simulink model "HMC"  (R2026a)
settings: Solver=ode1  StopTime=inf  FixedStep=0.0001
PreLoadFcn:
  | %load('C:\Users\bme_master\Desktop\mot\mot_6_deneme.mat')
  | 
  | 
  | %load('C:\Users\bme_master\Desktop\mot\PRE_G''s.mat')
PostLoadFcn:
  | , if any(exist('dsrtsu_mdlpostloadfcn', 'file') ~= 0), dsrtsu_mdlpostloadfcn('Execute', bdroot); end,
InitFcn:
  | %motor_control_init_m
  | %clear all
  | %close all
  | %clc
  | b=1e-8
  | StepSize = 1e-4;
  | N=1e-17;
  | 
  | VLV_0 =0;%120; %120
  | VA_0 = 0;%300; %300
  | VRV_0 = 0;%130;
  | VP_0 = 0;%500;
  | VLA_0 = 0;%20;
  | VV_0=5000;
  | VRA_0=0;
  | 
  | 
  | QLV_0 = 0;
  | QLA_0 = 0;
  | QP_0 = 0;
  | 
  | bh = 0;
  | th =0;
  | 
  | X_0 = [VLV_0 VA_0 VV_0 VP_0  VLA_0  VRA_0 VRV_0];
  | 
  | 
  | V0 = 10;
  | 
  | K1=.0004;%0.0001
  | K2=0.0009;%0.0009
  | KA=1;%1
  | C1=0.000000003;%0.0000003
  | lambda=6000;%3000
  | X_00 = [VLV_0 VA_0 VV_0 VRV_0];
  | 
  | r2 = 0.05/2;
  | A2 = pi*r2^2;
  | h2 = 0.63;
  | V2 = A2*h2;
  | 
  | 
  | r3 = 0.05/2;
  | A3 = pi*r3^2;
  | h3 = 0.63;
  | V3 = A3*h3;
  | 
  | 
  | rho = 997;
  | gg = 9.81;
  | %
  | init_min=0;
  | init_max=0;
  | %
  | PWM_Period =  StepSize;
  | PWM_Period_g1 = PWM_Period;
  | PWM_Period_g2 =PWM_Period;
  | PWM_Period_g3 = PWM_Period;
  | PWM_Period_g4 = PWM_Period;
  | PWM_Period_g5 = PWM_Period;
  | ... (+158 lines)
undefined symbols (not defined in the file or in its folder): Continuous, DiscIntNeverNeededParam, Time
libraries: powerlib_meascontrol x19, simulink x15, rti1202lib_adc_class1 x11, cstblocks x10, rti1202lib_dio_class1 x8, dspstat3 x3, rti1202lib_dac_class1 x1, dspswit3 x1, ctrlSharedLib x1, slpidlib x1, dsparch4 x1
(part 5 of 5)

== system HMC/Reference CVSs/eRV/RV_e_min/c_RV/PID ==
  s : Inport
  LTI System : cstblocks/LTI System  sys=tfa  IC=[]
  PID Controller : simulink/Continuous/PID Controller  Controller=PID  Form=Parallel  TimeDomain=Continuous-time  SampleTime=-1  IntegratorMethod=Forward Euler  FilterMethod=Forward Euler  ControllerParametersSource=internal  P=0  I=0.336541519886425  D=0  UseFilter=on  N=100  TunerSelectOption=Transfer Function Based (PID Tuner App)  InitialConditionSource=internal  InitialConditionForIntegrator=0  InitialConditionForFilter=0  DifferentiatorICPrevScaledInput=0  ExternalReset=none  TrackingMode=off  Kt=1  LimitOutput=off  UpperSaturationLimit=inf  LowerSaturationLimit=-inf  LinearizeAsGain=on  AntiWindupMode=none  Kb=1  POutMin=[]  POutMax=[]  IOutMin=[]  IOutMax=[]  DOutMin=[]  DOutMax=[]  NOutMin=[]  NOutMax=[]  SumOutMin=[]  SumOutMax=[]  SaturationOutMin=[]  SaturationOutMax=[]  PParamMin=[]  PParamMax=[]  IParamMin=[]  IParamMax=[]  DParamMin=[]  DParamMax=[]  NParamMin=[]  NParamMax=[]  KbParamMin=[]  KbParamMax=[]  KtParamMin=[]  KtParamMax=[]  KbOutMin=[]  KbOutMax=[]  KtOutMin=[]  KtOutMax=[]  IntegratorOutMin=[]  IntegratorOutMax=[]  FilterOutMin=[]  FilterOutMax=[]  SumI1OutMin=[]  SumI1OutMax=[]  SumI2OutMin=[]  SumI2OutMax=[]  SumI3OutMin=[]  SumI3OutMax=[]  SumI4OutMin=[]  SumI4OutMax=[]  SumDOutMin=[]  SumDOutMax=[]  DifferentiatorOutMin=[]  DifferentiatorOutMax=[]  FilterDiffOutCoefMin=[]  FilterDiffOutCoefMax=[]  ReciprocalOutMin=[]  ReciprocalOutMax=[]  SumDenOutMin=[]  SumDenOutMax=[]  SumNumOutMin=[]  SumNumOutMax=[]  DivideOutMin=[]  DivideOutMax=[]  IntegratorContinuousStateAttributes=''  IntegratorStateMustResolveToSignalObject=off  IntegratorRTWStateStorageClass=Auto  FilterContinuousStateAttributes=''  FilterStateMustResolveToSignalObject=off  FilterRTWStateStorageClass=Auto  ParallelPVariant=InternalParameters  IdealPVariant=Disabled  IVariant=InternalParameters  DVariant=InternalParameters  IntegratorVariant=Continuous  SatVariant=Disabled  AWVariant=Passthrough  PCopyVariant=Disabled  TRVariant=Disabled  FdbkBlocksVariant=Forward  IdealPFdbkVariant=Disabled  SatFdbkVariant=Disabled  DerivativeFilterVariant=ContFilter  NVariant=InternalParameters  NCopyVariant=Disabled  FilterICVariant=InternalICsFilter  IntegratorICVariant=InternalICs  ExternalResetVariant=Disabled  TRSumVariant=Passthrough  SumFdbkVariant=Disabled  SumVariant=Sum_PID
  Sum1 : Sum  Inputs=|+-
  To Workspace : ToWorkspace  VariableName=input  SampleTime=-1
  To Workspace1 : ToWorkspace  VariableName=output  SampleTime=-1
  E : Outport  VectorParamsAs1DForOutWhenUnconnected=off
  wires:
  LTI System/1 -> To Workspace1/1, E/1, Sum1/2
  Sum1/1 -> PID Controller/1
  s/1 -> Sum1/1
  PID Controller/1 -> LTI System/1, To Workspace/1

== system HMC/Reference CVSs/eRV/RV_e_min/real_c_RV/PID ==
  s : Inport
  LTI System : cstblocks/LTI System  sys=tfa  IC=[]
  PID Controller : simulink/Continuous/PID Controller  Controller=PID  Form=Parallel  TimeDomain=Continuous-time  SampleTime=-1  IntegratorMethod=Forward Euler  FilterMethod=Forward Euler  ControllerParametersSource=internal  P=0  I=0.336541519886425  D=0  UseFilter=on  N=100  TunerSelectOption=Transfer Function Based (PID Tuner App)  InitialConditionSource=internal  InitialConditionForIntegrator=0  InitialConditionForFilter=0  DifferentiatorICPrevScaledInput=0  ExternalReset=none  TrackingMode=off  Kt=1  LimitOutput=off  UpperSaturationLimit=inf  LowerSaturationLimit=-inf  LinearizeAsGain=on  AntiWindupMode=none  Kb=1  POutMin=[]  POutMax=[]  IOutMin=[]  IOutMax=[]  DOutMin=[]  DOutMax=[]  NOutMin=[]  NOutMax=[]  SumOutMin=[]  SumOutMax=[]  SaturationOutMin=[]  SaturationOutMax=[]  PParamMin=[]  PParamMax=[]  IParamMin=[]  IParamMax=[]  DParamMin=[]  DParamMax=[]  NParamMin=[]  NParamMax=[]  KbParamMin=[]  KbParamMax=[]  KtParamMin=[]  KtParamMax=[]  KbOutMin=[]  KbOutMax=[]  KtOutMin=[]  KtOutMax=[]  IntegratorOutMin=[]  IntegratorOutMax=[]  FilterOutMin=[]  FilterOutMax=[]  SumI1OutMin=[]  SumI1OutMax=[]  SumI2OutMin=[]  SumI2OutMax=[]  SumI3OutMin=[]  SumI3OutMax=[]  SumI4OutMin=[]  SumI4OutMax=[]  SumDOutMin=[]  SumDOutMax=[]  DifferentiatorOutMin=[]  DifferentiatorOutMax=[]  FilterDiffOutCoefMin=[]  FilterDiffOutCoefMax=[]  ReciprocalOutMin=[]  ReciprocalOutMax=[]  SumDenOutMin=[]  SumDenOutMax=[]  SumNumOutMin=[]  SumNumOutMax=[]  DivideOutMin=[]  DivideOutMax=[]  IntegratorContinuousStateAttributes=''  IntegratorStateMustResolveToSignalObject=off  IntegratorRTWStateStorageClass=Auto  FilterContinuousStateAttributes=''  FilterStateMustResolveToSignalObject=off  FilterRTWStateStorageClass=Auto  ParallelPVariant=InternalParameters  IdealPVariant=Disabled  IVariant=InternalParameters  DVariant=InternalParameters  IntegratorVariant=Continuous  SatVariant=Disabled  AWVariant=Passthrough  PCopyVariant=Disabled  TRVariant=Disabled  FdbkBlocksVariant=Forward  IdealPFdbkVariant=Disabled  SatFdbkVariant=Disabled  DerivativeFilterVariant=ContFilter  NVariant=InternalParameters  NCopyVariant=Disabled  FilterICVariant=InternalICsFilter  IntegratorICVariant=InternalICs  ExternalResetVariant=Disabled  TRSumVariant=Passthrough  SumFdbkVariant=Disabled  SumVariant=Sum_PID
  Sum1 : Sum  Inputs=|+-
  To Workspace : ToWorkspace  VariableName=input  SampleTime=-1
  To Workspace1 : ToWorkspace  VariableName=output  SampleTime=-1
  E : Outport  VectorParamsAs1DForOutWhenUnconnected=off
  wires:
  PID Controller/1 -> To Workspace/1, LTI System/1
  s/1 -> Sum1/1
  Sum1/1 -> PID Controller/1
  LTI System/1 -> Sum1/2, E/1, To Workspace1/1

== system HMC/IBS_LVAD/Subsystem1/Subsystem/eLV1/LV_e_min/Subsystem1 ==
  note: y = 0,0446x 2 - 6,3542x + 365,75
      | R² = 1
  Add18 : Sum
  Add19 : Sum
  Constant20 : Constant  Value=365.75
  Gain2 : Gain  Gain=0.0446
  Gain3 : Gain  Gain=- 6.3542
  Product15 : Product
  C_LV : Outport
  wires:
  Add18/1 -> Add19/1
  Gain3/1 -> Add18/2
  Product15/1 -> Gain2/1
  Constant20/1 -> Add19/2
  Gain2/1 -> Add18/1
  [HR] -> Product15/1, Product15/2, Gain3/1
  Add19/1 -> C_LV/1

== system HMC/IBS_LVAD/Subsystem1/Subsystem/eLV1/LV_e_min/Subsystem2 ==
  note: y = 0,0108x 2 - 4,2917x + 398,5
      | R² = 1
  note: y = 0,0011x 2 - 0,4292x + 39,85
      | R² = 1
  note: y = -0,0175x 2 + 5,625x - 264,5
      | R² = 1
  Add18 : Sum
  Add19 : Sum
  Constant20 : Constant  Value=398.5
  Gain : Gain  Gain=1/10000
  Gain2 : Gain  Gain=0.0108
  Gain3 : Gain  Gain=-4.2917
  Product15 : Product
  Scope : Scope
      settings: ActiveDisplayYMinimum=-0.00112  ActiveDisplayYMaximum=0.02012  DataLoggingVariableName=ScopeData2
  B_LV : Outport
  wires:
  Add18/1 -> Add19/1
  Gain3/1 -> Add18/2
  Product15/1 -> Gain2/1
  Constant20/1 -> Add19/2
  Gain2/1 -> Add18/1
  [HR] -> Product15/1, Product15/2, Gain3/1
  Add19/1 -> Gain/1
  Gain/1 -> Scope/1, B_LV/1

== system HMC/IBS_LVAD/Subsystem1/Subsystem/eLV1/LV_e_min/resting ==
  note: y = -4,3333x + 440
  Add19 : Sum
  Constant20 : Constant  Value=440
  Gain : Gain  Gain=1/10000
  Gain3 : Gain  Gain=-4.3333
  Scope : Scope
      settings: ActiveDisplayYMinimum=-0.00112  ActiveDisplayYMaximum=0.02012  DataLoggingVariableName=ScopeData2
  B_LV : Outport
  wires:
  Gain/1 -> B_LV/1, Scope/1
  Add19/1 -> Gain/1
  [insan] -> Gain3/1
  Constant20/1 -> Add19/2
  Gain3/1 -> Add19/1

== system HMC/IBS_LVAD/Subsystem1/Subsystem/eLV1/eLV1/PID ==
  s : Inport
  LTI System : cstblocks/LTI System  sys=tfa  IC=[]
  PID Controller : simulink/Continuous/PID Controller  Controller=PID  Form=Parallel  TimeDomain=Continuous-time  SampleTime=-1  IntegratorMethod=Forward Euler  FilterMethod=Forward Euler  ControllerParametersSource=internal  P=0  I=0.336541519886425  D=0  UseFilter=on  N=100  TunerSelectOption=Transfer Function Based (PID Tuner App)  InitialConditionSource=internal  InitialConditionForIntegrator=0  InitialConditionForFilter=0  DifferentiatorICPrevScaledInput=0  ExternalReset=none  TrackingMode=off  Kt=1  LimitOutput=off  UpperSaturationLimit=inf  LowerSaturationLimit=-inf  LinearizeAsGain=on  AntiWindupMode=none  Kb=1  POutMin=[]  POutMax=[]  IOutMin=[]  IOutMax=[]  DOutMin=[]  DOutMax=[]  NOutMin=[]  NOutMax=[]  SumOutMin=[]  SumOutMax=[]  SaturationOutMin=[]  SaturationOutMax=[]  PParamMin=[]  PParamMax=[]  IParamMin=[]  IParamMax=[]  DParamMin=[]  DParamMax=[]  NParamMin=[]  NParamMax=[]  KbParamMin=[]  KbParamMax=[]  KtParamMin=[]  KtParamMax=[]  KbOutMin=[]  KbOutMax=[]  KtOutMin=[]  KtOutMax=[]  IntegratorOutMin=[]  IntegratorOutMax=[]  FilterOutMin=[]  FilterOutMax=[]  SumI1OutMin=[]  SumI1OutMax=[]  SumI2OutMin=[]  SumI2OutMax=[]  SumI3OutMin=[]  SumI3OutMax=[]  SumI4OutMin=[]  SumI4OutMax=[]  SumDOutMin=[]  SumDOutMax=[]  DifferentiatorOutMin=[]  DifferentiatorOutMax=[]  FilterDiffOutCoefMin=[]  FilterDiffOutCoefMax=[]  ReciprocalOutMin=[]  ReciprocalOutMax=[]  SumDenOutMin=[]  SumDenOutMax=[]  SumNumOutMin=[]  SumNumOutMax=[]  DivideOutMin=[]  DivideOutMax=[]  IntegratorContinuousStateAttributes=''  IntegratorStateMustResolveToSignalObject=off  IntegratorRTWStateStorageClass=Auto  FilterContinuousStateAttributes=''  FilterStateMustResolveToSignalObject=off  FilterRTWStateStorageClass=Auto  ParallelPVariant=InternalParameters  IdealPVariant=Disabled  IVariant=InternalParameters  DVariant=InternalParameters  IntegratorVariant=Continuous  SatVariant=Disabled  AWVariant=Passthrough  PCopyVariant=Disabled  TRVariant=Disabled  FdbkBlocksVariant=Forward  IdealPFdbkVariant=Disabled  SatFdbkVariant=Disabled  DerivativeFilterVariant=ContFilter  NVariant=InternalParameters  NCopyVariant=Disabled  FilterICVariant=InternalICsFilter  IntegratorICVariant=InternalICs  ExternalResetVariant=Disabled  TRSumVariant=Passthrough  SumFdbkVariant=Disabled  SumVariant=Sum_PID
  Sum1 : Sum  Inputs=|+-
  To Workspace : ToWorkspace  VariableName=input  SampleTime=-1
  To Workspace1 : ToWorkspace  VariableName=output  SampleTime=-1
  E : Outport  VectorParamsAs1DForOutWhenUnconnected=off
  wires:
  LTI System/1 -> To Workspace1/1, E/1, Sum1/2
  Sum1/1 -> PID Controller/1
  s/1 -> Sum1/1
  PID Controller/1 -> LTI System/1, To Workspace/1

== system HMC/IBS_LVAD/Subsystem1/Subsystem/eRV1/RV_e_min/c_RV ==
  note: y = 0,0167x 2 - 3,3333x + 290
  Add18 : Sum
  Add19 : Sum
  Constant20 : Constant  Value=290
  Gain2 : Gain  Gain=0.0167
  Gain3 : Gain  Gain=-3.3333
  PID : Subsystem  Commented=on
  Product15 : Product
  Scope : Scope
      settings: ActiveDisplayYMinimum=1.07059  ActiveDisplayYMaximum=1.42514
  Stair Generator : powerlib_meascontrol/Pulse & Signal Generators/Stair Generator  Commented=on  t=[0,50,100,150]  e=[3.25,3.5,3.75,4]  Ts=stepsize
      settings: SourceProductName=Simscape Electrical
  Stair Generator1 : powerlib_meascontrol/Pulse & Signal Generators/Stair Generator  Commented=on  t=[100,200,300,400]  e=[3.25,3.5,3.75,4]  Ts=stepsize
      settings: SourceProductName=Simscape Electrical
  Output : Outport
  wires:
  Stair Generator1/1 -> PID/1(s)
  Gain2/1 -> Add18/1
  Gain3/1 -> Add18/2
  [HR] -> Product15/1, Product15/2, Gain3/1
  Add18/1 -> Add19/1
  Product15/1 -> Gain2/1
  Constant20/1 -> Add19/2
  Add19/1 -> Scope/1, Output/1

== system HMC/IBS_LVAD/Subsystem1/Subsystem/eRV1/Subsystem2/k_0 ==
  note: y = -0,0042x 2 - 0,0417x + 257,5
      | R² = 1
  In1 : Inport
  Add4 : Sum
  Add5 : Sum
  Constant4 : Constant  Value=257.5
  Gain : Gain  Gain=-0.0041
  Gain1 : Gain  Gain=-0.0417
  Multiply : Gain  Gain=1/1000
  Product8 : Product
  Out1 : Outport
  wires:
  Add4/1 -> Add5/1
  In1/1 -> Gain1/1, Product8/2, Product8/1
  Product8/1 -> Gain/1
  Gain1/1 -> Add4/2
  Gain/1 -> Add4/1
  Constant4/1 -> Add5/2
  Add5/1 -> Multiply/1
  Multiply/1 -> Out1/1

== system HMC/IBS_LVAD/Subsystem1/Subsystem/eRV1/Subsystem2/k_1 ==
  note: y = 0,0158x 2 - 5,0417x + 445,5
      | R² = 1
  In1 : Inport
  Add6 : Sum
  Add7 : Sum
  Constant7 : Constant  Value=445.5
  Gain2 : Gain  Gain=0.0158
  Gain3 : Gain  Gain=-5.0417
  Multiply : Gain  Gain=1/1000
  Product10 : Product
  Out1 : Outport
  wires:
  Constant7/1 -> Add7/2
  Gain2/1 -> Add6/1
  In1/1 -> Gain3/1, Product10/2, Product10/1
  Gain3/1 -> Add6/2
  Add6/1 -> Add7/1
  Product10/1 -> Gain2/1
  Add7/1 -> Multiply/1
  Multiply/1 -> Out1/1

== system HMC/IBS_LVAD/Subsystem1/Subsystem/eRV1/eRV2/PID ==
  s : Inport
  LTI System : cstblocks/LTI System  sys=tfa  IC=[]
  PID Controller : simulink/Continuous/PID Controller  Controller=PID  Form=Parallel  TimeDomain=Continuous-time  SampleTime=-1  IntegratorMethod=Forward Euler  FilterMethod=Forward Euler  ControllerParametersSource=internal  P=0  I=0.336541519886425  D=0  UseFilter=on  N=100  TunerSelectOption=Transfer Function Based (PID Tuner App)  InitialConditionSource=internal  InitialConditionForIntegrator=0  InitialConditionForFilter=0  DifferentiatorICPrevScaledInput=0  ExternalReset=none  TrackingMode=off  Kt=1  LimitOutput=off  UpperSaturationLimit=inf  LowerSaturationLimit=-inf  LinearizeAsGain=on  AntiWindupMode=none  Kb=1  POutMin=[]  POutMax=[]  IOutMin=[]  IOutMax=[]  DOutMin=[]  DOutMax=[]  NOutMin=[]  NOutMax=[]  SumOutMin=[]  SumOutMax=[]  SaturationOutMin=[]  SaturationOutMax=[]  PParamMin=[]  PParamMax=[]  IParamMin=[]  IParamMax=[]  DParamMin=[]  DParamMax=[]  NParamMin=[]  NParamMax=[]  KbParamMin=[]  KbParamMax=[]  KtParamMin=[]  KtParamMax=[]  KbOutMin=[]  KbOutMax=[]  KtOutMin=[]  KtOutMax=[]  IntegratorOutMin=[]  IntegratorOutMax=[]  FilterOutMin=[]  FilterOutMax=[]  SumI1OutMin=[]  SumI1OutMax=[]  SumI2OutMin=[]  SumI2OutMax=[]  SumI3OutMin=[]  SumI3OutMax=[]  SumI4OutMin=[]  SumI4OutMax=[]  SumDOutMin=[]  SumDOutMax=[]  DifferentiatorOutMin=[]  DifferentiatorOutMax=[]  FilterDiffOutCoefMin=[]  FilterDiffOutCoefMax=[]  ReciprocalOutMin=[]  ReciprocalOutMax=[]  SumDenOutMin=[]  SumDenOutMax=[]  SumNumOutMin=[]  SumNumOutMax=[]  DivideOutMin=[]  DivideOutMax=[]  IntegratorContinuousStateAttributes=''  IntegratorStateMustResolveToSignalObject=off  IntegratorRTWStateStorageClass=Auto  FilterContinuousStateAttributes=''  FilterStateMustResolveToSignalObject=off  FilterRTWStateStorageClass=Auto  ParallelPVariant=InternalParameters  IdealPVariant=Disabled  IVariant=InternalParameters  DVariant=InternalParameters  IntegratorVariant=Continuous  SatVariant=Disabled  AWVariant=Passthrough  PCopyVariant=Disabled  TRVariant=Disabled  FdbkBlocksVariant=Forward  IdealPFdbkVariant=Disabled  SatFdbkVariant=Disabled  DerivativeFilterVariant=ContFilter  NVariant=InternalParameters  NCopyVariant=Disabled  FilterICVariant=InternalICsFilter  IntegratorICVariant=InternalICs  ExternalResetVariant=Disabled  TRSumVariant=Passthrough  SumFdbkVariant=Disabled  SumVariant=Sum_PID
  Sum1 : Sum  Inputs=|+-
  To Workspace : ToWorkspace  VariableName=input  SampleTime=-1
  To Workspace1 : ToWorkspace  VariableName=output  SampleTime=-1
  E : Outport  VectorParamsAs1DForOutWhenUnconnected=off
  wires:
  PID Controller/1 -> To Workspace/1, LTI System/1
  s/1 -> Sum1/1
  Sum1/1 -> PID Controller/1
  LTI System/1 -> Sum1/2, E/1, To Workspace1/1

== system HMC/IBS_LVAD/Subsystem1/Subsystem/eRV1/RV_e_min/c_RV/PID ==
  s : Inport
  LTI System : cstblocks/LTI System  sys=tfa  IC=[]
  PID Controller : simulink/Continuous/PID Controller  Controller=PID  Form=Parallel  TimeDomain=Continuous-time  SampleTime=-1  IntegratorMethod=Forward Euler  FilterMethod=Forward Euler  ControllerParametersSource=internal  P=0  I=0.336541519886425  D=0  UseFilter=on  N=100  TunerSelectOption=Transfer Function Based (PID Tuner App)  InitialConditionSource=internal  InitialConditionForIntegrator=0  InitialConditionForFilter=0  DifferentiatorICPrevScaledInput=0  ExternalReset=none  TrackingMode=off  Kt=1  LimitOutput=off  UpperSaturationLimit=inf  LowerSaturationLimit=-inf  LinearizeAsGain=on  AntiWindupMode=none  Kb=1  POutMin=[]  POutMax=[]  IOutMin=[]  IOutMax=[]  DOutMin=[]  DOutMax=[]  NOutMin=[]  NOutMax=[]  SumOutMin=[]  SumOutMax=[]  SaturationOutMin=[]  SaturationOutMax=[]  PParamMin=[]  PParamMax=[]  IParamMin=[]  IParamMax=[]  DParamMin=[]  DParamMax=[]  NParamMin=[]  NParamMax=[]  KbParamMin=[]  KbParamMax=[]  KtParamMin=[]  KtParamMax=[]  KbOutMin=[]  KbOutMax=[]  KtOutMin=[]  KtOutMax=[]  IntegratorOutMin=[]  IntegratorOutMax=[]  FilterOutMin=[]  FilterOutMax=[]  SumI1OutMin=[]  SumI1OutMax=[]  SumI2OutMin=[]  SumI2OutMax=[]  SumI3OutMin=[]  SumI3OutMax=[]  SumI4OutMin=[]  SumI4OutMax=[]  SumDOutMin=[]  SumDOutMax=[]  DifferentiatorOutMin=[]  DifferentiatorOutMax=[]  FilterDiffOutCoefMin=[]  FilterDiffOutCoefMax=[]  ReciprocalOutMin=[]  ReciprocalOutMax=[]  SumDenOutMin=[]  SumDenOutMax=[]  SumNumOutMin=[]  SumNumOutMax=[]  DivideOutMin=[]  DivideOutMax=[]  IntegratorContinuousStateAttributes=''  IntegratorStateMustResolveToSignalObject=off  IntegratorRTWStateStorageClass=Auto  FilterContinuousStateAttributes=''  FilterStateMustResolveToSignalObject=off  FilterRTWStateStorageClass=Auto  ParallelPVariant=InternalParameters  IdealPVariant=Disabled  IVariant=InternalParameters  DVariant=InternalParameters  IntegratorVariant=Continuous  SatVariant=Disabled  AWVariant=Passthrough  PCopyVariant=Disabled  TRVariant=Disabled  FdbkBlocksVariant=Forward  IdealPFdbkVariant=Disabled  SatFdbkVariant=Disabled  DerivativeFilterVariant=ContFilter  NVariant=InternalParameters  NCopyVariant=Disabled  FilterICVariant=InternalICsFilter  IntegratorICVariant=InternalICs  ExternalResetVariant=Disabled  TRSumVariant=Passthrough  SumFdbkVariant=Disabled  SumVariant=Sum_PID
  Sum1 : Sum  Inputs=|+-
  To Workspace : ToWorkspace  VariableName=input  SampleTime=-1
  To Workspace1 : ToWorkspace  VariableName=output  SampleTime=-1
  E : Outport  VectorParamsAs1DForOutWhenUnconnected=off
  wires:
  LTI System/1 -> To Workspace1/1, E/1, Sum1/2
  Sum1/1 -> PID Controller/1
  s/1 -> Sum1/1
  PID Controller/1 -> LTI System/1, To Workspace/1

== matlab function HMC/Compressor to P1 Fill ==
  data: error input; Measured_Delta_P input; input_Current output; Q_Calculated input; difference input
function input_Current   = Valve_Current_Calculator_1_6(error, Measured_Delta_P, Q_Calculated,difference)

a1 =       154.5;
a2 =           0;
b1 =         166;
c1 =       74.85;
c2 =           0;

y = Measured_Delta_P;
z = Q_Calculated;

if(error > 0)
    
%     if (difference >= 0)
%         [minDistanceQ, indexOfQ] = min( abs( Q_increase_1_6(indexOfDP,:) - Q_Calculated ) );
%     else
%         [minDistanceQ, indexOfQ] = min( abs( Q_decrease_1_6(indexOfDP,:) - Q_Calculated ) );
%     end
%     
   
    input_Current = real(b1 - sqrt(complex((c1*y + c2)^2*log(complex((a1*y + a2)/z)))));
   
else
    input_Current = 0;
end

== matlab function HMC/P2 Fill ==
  data: error input; Measured_Delta_P input; input_Current output; Q_Calculated input; difference input
function input_Current = Valve_Current_Calculator_4_0(error, Measured_Delta_P, Q_Calculated, difference)


a1 =       580.9;
a2 =       3.908;
b1 =         166;
c1 =       328.3;
c2 =       5.419;

y = Measured_Delta_P;
z = Q_Calculated;

if(error > 0)
   
%     if (difference >= 0)
%         [minDistanceQ, indexOfQ] = min( abs( Q_increase_0_4(indexOfDP,:) - Q_Calculated ) );
%     else
%         [minDistanceQ, indexOfQ] = min( abs( Q_decrease_0_4(indexOfDP,:) - Q_Calculated ) );
%     end
    
    input_Current = real(b1 - sqrt(complex((c1*y + c2)^2*log(complex((a1*y + a2)/z)))));
else
    input_Current = 0;
end

== matlab function HMC/MATLAB Function4 ==
  data: u input; y output
function y = fcn(u)
a =     0.0046;
b =      0.0408;

if u <=0
    y = 0;
else
    y = a*u+b;
end


% function y = fcn(u)
% a =     0.05866;
% b =      0.5277;
% y = a*u^b;

== matlab function HMC/MATLAB Function5 ==
  data: u input; y output
function y = fcn(u)
a =     0.0046;
b =      0.0408;

if u <=0
    y = 0;
else
    y = a*u+b;
end


% function y = fcn(u)
% a =     0.05866;
% b =      0.5277;
% y = a*u^b;

== matlab function HMC/P2 Release ==
  data: error input; Measured_Delta_P input; input_Current output; Q_Calculated input; difference input
function input_Current   = Valve_Current_Calculator_4_0(error, Measured_Delta_P, Q_Calculated, difference)


a1 =       580.9;
a2 =       3.908;
b1 =         190;
c1 =       328.3;
c2 =       5.419;

y = Measured_Delta_P;
z = Q_Calculated;

if(error < 0)
   
%     if (difference >= 0)
%         [minDistanceQ, indexOfQ] = min( abs( Q_increase_0_4(indexOfDP,:) - Q_Calculated ) );
%     else
%         [minDistanceQ, indexOfQ] = min( abs( Q_decrease_0_4(indexOfDP,:) - Q_Calculated ) );
%     end
    
    input_Current = real(b1 - sqrt(complex((c1*y + c2)^2*log(complex((a1*y + a2)/z)))));
else
    input_Current = 0;
end

== matlab function HMC/MATLAB Function2 ==
  data: y_kalman_in input; P_kalman_in input; Qk input; Rk input; Pc input; z_meas input; Pvac input; Qp input; Qs input; dt input; ref input; ref_pre input; K_Lya input; Ugp input; kalman_z2 input; y_kalman_out output; P_kalman_out output; G output; Er output; VS input
function [y_kalman_out,P_kalman_out,G,Er] = fcn(y_kalman_in,P_kalman_in,Qk,Rk,Pc,z_meas, Pvac,Qp,Qs,dt,ref,ref_pre,K_Lya,Ugp,kalman_z2, VS)
%% Signal Demux

P1 = y_kalman_in(1);  % Air pressure reduction tank
P2p = y_kalman_in(2); % Aorta tank air pressure
P2 = y_kalman_in(3);  % Aorta tank total pressure
P3 = y_kalman_in(4);  % LV tank total pressure
P3p = y_kalman_in(5); % LV tank air pressure
Qgp = y_kalman_in(6); % Gear pump flow
Qvad = y_kalman_in(7);
Qsp = y_kalman_in(8);


P1_z2 = kalman_z2(1);  % Air pressure reduction tank
P2p_z2 = kalman_z2(2); % Aorta tank air pressure
P2_z2 = kalman_z2(3);  % Aorta tank total pressure
P3_z2 = kalman_z2(4);  % LV tank total pressure
P3p_z2 = kalman_z2(5); % LV tank air pressure
Qgp_z2 = kalman_z2(6); % Gear pump flow
Qvad_z2 = kalman_z2(7);
Qsp_z2 = kalman_z2(8);

%%
% load('C:\Users\bme_master\Desktop\sys_id\tf\gp_tf_28_12.mat')
% load('C:\Users\bme_master\Desktop\sys_id\tf\updated_gp_tfsComp.mat')
% [A1,B1,C1,D1]=tf2ss(tf8_4.Numerator{1},tf8_4.Denominator{1});
% [A2,B2,C2,D2]=tf2ss(tf8_4.Numerator{2},tf8_4.Denominator{2});
% ssgp1=ss(A1,B1,C1,D1);
% ssgp2=ss(A2,B2,C2,D2);
% csysgp1=canon(ssgp1,'companion');
% csysgp2=canon(ssgp2,'companion');

P1ref = ref(1);
P2ref = ref(2);
P3ref = ref(3);

P1ref_pre = ref_pre(1);
P2ref_pre = ref_pre(2);
P3ref_pre = ref_pre(3);

K1 = K_Lya(1);
K_Ao_in = K_Lya(2);
K_Ao_out = K_Lya(3);
K_LV_in = K_Lya(4);
K_LV_out = K_Lya(5);

Qin2 = Qp;
Qout2 = Qs;
Qin3 = Qs;
Qout3 = Qp;

% w_gp = GP_VAD(1);
% i_gp = GP_VAD(2);


%% System Constants
R = 287;
T = 273+23;

r1 = 0.09/2;
A1 = pi*r1^2;
h1 = 0.1;
V1 = A1*h1;

r2 = 0.085/2;
A2 = pi*r2^2;
h2 = 0.200;
V2 = A2*h2;

r3 = 0.085/2;
A3 = pi*r3^2;
h3 = 0.200;
V3 = A3*h3;

rho = 997;
g = 9.81;
eh2 = rho*g/A2;
eh3 = rho*g/A3;

L_gp = 1.44*(10^-3); % H
R_gp = 0.48;% ohm
R_bf = 2.399e9; % Pa s/m^3
K_gp_emf = 72.4*(10^-3); % V s
K_gp_T = K_gp_emf; % V s
J_gp = 0.293*(10^-3); % kg m^2

l = 0.025;% m
r0 = 0.017; ri = 0.012; % m 
V_gp_SV = 1.59e-6; % m^3/rad
tr0 = 0.3*10^-3; % N
tr1 = 44.9*10^-6; % N s/m

%% Errors
E1 = P1ref-P1;
E_Ao = P2ref-P2;
E_Lv = P3ref-P3;
Er = [E1 E_Ao E_Lv]';

%% Derivatives
P1ref_dot = (P1ref-P1ref_pre)/dt;
P2ref_dot = (P2ref-P2ref_pre)/dt;
P3ref_dot = (P3ref-P3ref_pre)/dt;

%% Admitance  Calc New 20/09/2022
% Aorta 

g_Ao_in = ((P2p - (P2 - eh2*V2))/(eh2*R*T*(P1 - P2p)))*(P2ref_dot-K_Ao_in*E_Ao);

g_Ao_in = g_Ao_in*VS;

g_Ao_out = (K_Ao_out*E_Ao)*(P2p - (P2 - eh2*V2))/((eh2*R*T*(P2p - Pvac))) + (eh2*(2*P2p - (P2 - eh2*V2))*(Qin2-Qout2)/(eh2*R*T*(P2p - Pvac))); 

g_Ao_out = g_Ao_out*VS ; 
%LV

g_LV_in= ((P3p - (P3 - eh3*V3))/(eh3*R*T*(P1 - P3p)))*(P3ref_dot-K_LV_in*E_Lv);
g_LV_in = g_LV_in*VS;

g_LV_out= (K_LV_out*E_Lv)*(P3p - (P3 - eh3*V3))/((eh3*R*T*(P3p - Pvac))) + (eh3*(2*P3p - (P3 - eh3*V3))*(Qin3-Qout3)/(eh3*R*T*(P3p - Pvac))); 
g_LV_out = g_LV_out*VS ;
% P1 tank

g1 = V1/(R*T*(Pc-P1))*(P1ref_dot-K1*E1 + g_Ao_in*(R*T*(P1-P2p))/V1 + g_LV_in*(R*T*(P1-P3p))/V1);
g1 = g1*VS; 

G = [g1 g_Ao_in g_Ao_out g_LV_in g_LV_out]';

%% Precalculations for Kalman

% P1_dot_eq = (((R*T)/V1)*((g1*(Pc-P1)-g_Ao_in*(P1-P2p)-g_LV_in*(P1-P3p))));

%% P2p P2
AA2 = g_Ao_in*(P1-P2p)-g_Ao_out*(P2p-Pvac);
BB2 = (eh2*V2-(P2-P2p))/(eh2);
CC2 = (P2p/BB2)*(Qin2-Qout2);

P2_dot_eq = R*T*(AA2/BB2)+((2*P2p-(P2-eh2*V2))/BB2)*(Qin2-Qout2);
P2p_dot_eq = R*T*(AA2/BB2) + CC2;
%% P3p P3 
AA3 = g_LV_in*(P1-P3p)-(g_LV_out*2)*(P3p-Pvac);
BB3 = (eh3*V3-(P3-P3p))/(eh3);
CC3 = (P3p/BB3)*(Qin3-Qout3);

P3_dot_eq = R*T*(AA3/BB3)+((2*P3p-(P3-eh3*V3))/BB3)*(Qin3-Qout3);
P3p_dot_eq = R*T*(AA3/BB3) + CC3 ;

%% Discrete State Marices

A = eye(8);
Bu = zeros(8,1);

% Bu(1) =(P1-P1_z2)*dt; %P1_dot_eq*dt; %P1
% Bu(2) = (P2p-P2p_z2)*dt; %P2p_dot_eq*dt %P2p
% Bu(3) = (P2-P2_z2)*dt; %P2_dot_eq*dt %P2
% Bu(4) = (P3-P3_z2)*dt; %P3_dot_eq*dt %P3
% Bu(5) = (P3p-P3p_z2)*dt; %P3p_dot_eq*dt %P3p
% Bu(6) = (Qgp-Qgp_z2)*dt; %Qgp
% Bu(7) = (Qvad-Qvad_z2)*dt; %Qvad

Bu(1) =(P1-P1_z2)*dt; %P1
Bu(2) =P2p_dot_eq*dt; %P2p
Bu(3) =P2_dot_eq*dt; %P2
Bu(4) =P3_dot_eq*dt; %P3
Bu(5) =P3p_dot_eq*dt; %P3p
Bu(6) =(Qgp-Qgp_z2)*dt;%Qgp
Bu(7) =(Qvad-Qvad_z2)*dt; %Qvad
Bu(8) =(Qsp-Qsp_z2)*dt; %Qsp

H = eye(8);

%% Kalman Filter
y_pred = A*y_kalman_in +Bu;
P_pred = A*P_kalman_in*A' + Qk;

Kk = P_kalman_in*H'*(H*P_kalman_in*H'+Rk)^-1;

y_kalman_out = zeros(8,1);
P_kalman_out = zeros(8);

y_kalman_out = y_pred+Kk*(z_meas-H*y_pred); 
P_kalman_out = P_pred-Kk*H*P_pred;

== matlab function HMC/MATLAB Function6 ==
  data: Qk output; Rk output; Qk_gain input; Rk_gain input
function [Qk,Rk] = fcn(Qk_gain,Rk_gain)

Qk = zeros(8);
Qk = diag(Qk_gain);
%Qk(1:5,1:5) = Qk_gain(1:5)*Qk_gain(1:5)';

Rk = zeros(8);
Rk_diag = diag(Rk_gain);
Rk = Rk_diag;

== matlab function HMC/MATLAB Function7 ==
  data: u input; y output
function y = fcn(u)
a =     0.0046;
b =      0.0408;

if u <=0
    y = 0;
else
    y = a*u+b;
end


% function y = fcn(u)
% a =     0.05866;
% b =      0.5277;
% y = a*u^b;

== matlab function HMC/MATLAB Function8 ==
  data: u input; y output
function y = fcn(u)
a =     0.0046;
b =      0.0408;

if u <=0
    y = 0;
else
    y = a*u+b;
end


% function y = fcn(u)
% a =     0.05866;
% b =      0.5277;
% y = a*u^b;

== matlab function HMC/P3 Fill ==
  data: error input; Measured_Delta_P input; input_Current output; Q_Calculated input; difference input
function input_Current = Valve_Current_Calculator_4_0(error, Measured_Delta_P, Q_Calculated, difference)


a1 =       580.9;
a2 =       3.908;
b1 =         166;
c1 =       328.3;
c2 =       5.419;

y = Measured_Delta_P;
z = Q_Calculated;

if(error > 0)
   
%     if (difference >= 0)
%         [minDistanceQ, indexOfQ] = min( abs( Q_increase_0_4(indexOfDP,:) - Q_Calculated ) );
%     else
%         [minDistanceQ, indexOfQ] = min( abs( Q_decrease_0_4(indexOfDP,:) - Q_Calculated ) );
%     end
    
    input_Current = real(b1 - sqrt(complex((c1*y + c2)^2*log(complex((a1*y + a2)/z)))));
else
    input_Current = 0;
end

== matlab function HMC/P3 Release ==
  data: error input; Measured_Delta_P input; input_Current output; Q_Calculated input; difference input
function input_Current   = Valve_Current_Calculator_4_0(error, Measured_Delta_P, Q_Calculated, difference)


a1 =       580.9;
a2 =       3.908;
b1 =         190;
c1 =       328.3;
c2 =       5.419;

y = Measured_Delta_P;
z = Q_Calculated;

if(error < 0)
   
%     if (difference >= 0)
%         [minDistanceQ, indexOfQ] = min( abs( Q_increase_0_4(indexOfDP,:) - Q_Calculated ) );
%     else
%         [minDistanceQ, indexOfQ] = min( abs( Q_decrease_0_4(indexOfDP,:) - Q_Calculated ) );
%     end
    
    input_Current = real(b1 - sqrt(complex((c1*y + c2)^2*log(complex((a1*y + a2)/z)))));
else
    input_Current = 0;
end

== matlab function HMC/KALMAN 3 STATES PLA/MATLAB Function1 ==
  data: u input; y output; plv input; pla input
function y = fcn(u,plv,pla)

elv=u(1);
elv_dot=u(2);
glv=u(3);
ea=u(4);
ga=u(5);
ela=u(6);


if pla >= plv
gla=u(7);
else
gla=0;
end
 y=[-ea*glv-ea*ga,ea*glv,ea*ga;
 glv*elv,-(elv_dot/elv)-gla*elv-glv*elv,gla*elv;
 ela*ga,gla*ela,-ela*ga-gla*ela];

== matlab function HMC/Reference CVSs/Pressures Flows and Volumes/MATLAB Function ==
  data: u input; y output; HR input
function y = fcn(u,HR)

tbeatlol =60/HR;
y = mod(u,tbeatlol);
end

== matlab function HMC/KALMAN 3 STATES PLA/MATLAB Function9 ==
  data: u input; y output
function y = fcn(u)

elv=u(1);
elv_dot=u(2);
glv=u(3);
ea=u(4);
gao=u(5);
ela=u(6);
gla=u(7);


y =[0;-elv_dot;0];

== matlab function HMC/Reference CVSs/Pressures Flows and Volumes/Subsystem5/VolumesForVAD/MATLAB Function ==
  data: u input; y output; HR input
function y = fcn(u,HR)

tbeatlol =60/HR;
y = mod(u,tbeatlol);
end

== matlab function HMC/Subsystem/MATLAB Function ==
  data: u input; lol output; delayed_u input; pre_bob input
function lol  = fcn(u,delayed_u,pre_bob)



bob = u-delayed_u


if bob ~= 0 
    
    lol = bob
else
    
    lol = pre_bob
end

== matlab function HMC/Subsystem/MATLAB Function1 ==
  data: d_1 input; y output; d_2 input; d_3 input; d_4 input; d_5 input; ty input
function y  = fcn(d_1,d_2,d_3,d_4,d_5,ty)


b = [d_1,d_2,d_3,d_4,d_5];
c= find(b==d_5);
d=length(c);

 if d >=3
    y= d_5;
    
 else 
     y=ty;
 end

== matlab function HMC/Subsystem/MATLAB Function10 ==
  data: time input; th output; on_off input; tpr input
function th = fcn(time,on_off,tpr)



%30 
if on_off == 1 
    th = time;
    a=0;
else
    th= tpr
    a=1;
end

== matlab function HMC/Real_IBS/MATLAB Function1 ==
  data: alpha_Q input; v output; alpha_P input; J input; lambda input; KV input; kv input; DP input; Q_vad_dot input; EV input; EV_int input; K3 input; K4 input; DV_dot_ref input; Q_vad input; Q_gp input; A input
function v  = fcn(alpha_Q,alpha_P,J,lambda,KV,kv,DP,Q_vad_dot,EV,EV_int,K3,K4,DV_dot_ref,Q_vad,Q_gp,A)



% A=((KV*(K3-kv))/2*alpha_Q);
% B=(KV+K4*(KV^2-lambda)/(4*alpha_Q^2));
% C= J/kv;
% D= (J/(alpha_Q*kv))*Q_vad_dot;
% E= (alpha_P/kv)*DP;
% e_w = (1/(2*alpha_Q))*(-KV*EV-lambda*EV_int-DV_dot_ref+2*Q_vad)-(Q_gp/alpha_Q);
% 
% 
% 
% y = C*(A+B*e_w)+(D+E);

EQ = Q_vad - Q_gp ;

A1 = alpha_P/kv;
A2 = J/(kv*alpha_Q);
A3 = (J/kv)*((KV/alpha_Q)+ (K4*(KV^2 - lambda))/(4*alpha_Q^3)); 
A4 = ((-J)/(2*alpha_Q*kv))*(KV^2 + (K3*K4*(KV^2 - lambda))/(4*alpha_Q^2));

A1 = A(1);
A2 = A(2);
A3 = A(3);
A4 = A(4);


v = A1*DP + A2*Q_vad_dot + A3*EQ + A4*EV;

== matlab function HMC/IBS_LVAD/Subsystem1/MATLAB Function1 ==
  data: K1 input; w output; Qvad_ref output; K2 input; KA input; C1 input; lambda input; PLV input; PA input; PV input; PRA input; QLA input; QLV input; QA input; QV input; QRA input; Qvad input; VLV input; eRA input; eA input; eV input; eLV input; eLV_dot input; gA input; gV input; gLV input; QA_ref input; QA_ref_dot input; QA_ref_ddot input; EQs output; S output
function [w ,Qvad_ref,EQs,S]  = fcn(K1, K2, KA, C1, lambda, PLV, PA, PV, PRA, QLA, QLV, QA, QV, QRA, Qvad, VLV, eRA, eA, eV, eLV, eLV_dot, gA, gV, gLV, QA_ref, QA_ref_dot, QA_ref_ddot)

% function [w ,Qvad_ref, TT,TTT]  = fcn(K1, K2, KA, C1, lambda, PLV, PA, PV, PRA, QLA, QLV, QA, QV, QRA, Qvad, VLV, eRA, eA, eV, eLV, eLV_dot, gA, gV, gLV, QA_ref, QA_ref_dot, QA_ref_ddot)

%% constants
ck = 16.66666;

alpha=3.683;%e-6;
a1=4.414e-05/(ck^2);
a2=-1.413/(ck^2);
b1=0.0007747/ck;
b2=-0.8314/ck;

L=6*(1000/(60^2));

%% P_dot
PLV_dot=eLV*(QLA-QLV-Qvad) + eLV_dot*VLV;
PA_dot=eA*(QLV+Qvad-QA);
PV_dot=eV*(QA-QV);
PRA_dot=eRA*(QV-QRA);


%% Q_Dot
QLV_dot =gLV*(PLV_dot-PA_dot); 
QA_dot = gA*(PA_dot-PV_dot);
QV_dot = gV*(PV_dot-PRA_dot);

%% 

S=((4*C1*QLV*alpha*eA^2*gA^2 + C1*Qvad^4*a1^2*eA^2*gA^2*gLV + C1*Qvad^2*b1^2*eA^2*gA^2*gLV + 4*K2*L*QA_ref_dot*alpha*gLV*lambda - 4*C1^2*KA*L*QA_ref_dot*alpha*gLV - 4*C1*Qvad^2*a2*alpha*eA^2*gA^2*gLV + 2*C1*Qvad^3*a1*b1*eA^2*gA^2*gLV + 4*C1*L*QA_dot*alpha*eA^2*gA^2*gLV - 4*C1*L*QLV_dot*alpha*eA^2*gA^2*gLV - 4*C1*Qvad*alpha*b2*eA^2*gA^2*gLV - 4*K1*K2*L*QA*alpha*gLV*lambda + 4*K1*K2*L*QA_ref*alpha*gLV*lambda + 4*C1*L*QA_ref_ddot*alpha*eA*gA*gLV + 4*C1^2*K1*KA*L*QA*alpha*gLV - 4*C1^2*K1*KA*L*QA_ref*alpha*gLV + 4*K2*L*QA*alpha*eA*gA*gLV*lambda - 4*K2*L*QLV*alpha*eA*gA*gLV*lambda + 4*K2*L*QA*alpha*eV*gA*gLV*lambda - 4*K2*L*QV*alpha*eV*gA*gLV*lambda - 4*K2*L*Qvad*alpha*eA*gA*gLV*lambda - 4*C1^2*KA*L*QA*alpha*eA*gA*gLV + 4*C1^2*KA*L*QLV*alpha*eA*gA*gLV - 4*C1^2*KA*L*QA*alpha*eV*gA*gLV + 4*C1^2*KA*L*QV*alpha*eV*gA*gLV + 4*C1^2*KA*L*Qvad*alpha*eA*gA*gLV + 4*C1*L*QA_dot*alpha*eA*eV*gA^2*gLV - 4*C1*L*QV_dot*alpha*eA*eV*gA^2*gLV + 4*C1*K1*KA*L*QA*alpha*eA*gA*gLV - 4*C1*K1*KA*L*QA_ref*alpha*eA*gA*gLV)/(C1*gLV));
S =max(0,S);

w=(+S^(1/2) - Qvad^2*a1*eA*gA - Qvad*b1*eA*gA)/(2*alpha*eA*gA);

% w = 3; 

EQ1=((K1)/(gA*eA))*QA_ref;
EQ2=-((K1)/(gA*eA))*QA;
EQ3=(1/gA*eA)*QA_ref_dot;
EQ4=-QLV+((eV+eA)/eA)*QA;
EQ5=-(eV/eA)*QV;
EQ6=0;
EQs=[EQ1 EQ2 EQ3 EQ4 EQ5 EQ6]';
Qvad_ref=EQ1+EQ2+EQ3+EQ4+EQ5+EQ6;
 

% 
% G1=+ (4*QLV*alpha*eA^2*gA^2)/gLV; 
% G2=+Qvad^4*a1^2*eA^2*gA^2;
% G3=+Qvad^2*b1^2*eA^2*gA^2;
% G4=+ (4*K2*L*QA_ref_dot*alpha*lambda)/C1 ;
% G5=- 4*C1*KA*L*QA_ref_dot*alpha;
% G6=- 4*Qvad^2*a2*alpha*eA^2*gA^2;
% G7=+ 2*Qvad^3*a1*b1*eA^2*gA^2;
% G8=+ 4*L*QA_dot*alpha*eA^2*gA^2;
% G9=- 4*L*QLV_dot*alpha*eA^2*gA^2;
% G10=- 4*Qvad*alpha*b2*eA^2*gA^2;
% G11=- (4*K1*K2*L*QA*alpha*lambda)/C1;
% G12=+ (4*K1*K2*L*QA_ref*alpha*lambda)/C1;
% G13=+ 4*L*QA_ref_ddot*alpha*eA*gA;
% G14=+ 4*C1*K1*KA*L*QA*alpha;
% G15=- 4*C1*K1*KA*L*QA_ref*alpha;
% G16=+ (4*K2*L*QA*alpha*eA*gA*lambda)/C1;
% G17=- (4*K2*L*QLV*alpha*eA*gA*lambda)/C1;
% G18=+ (4*K2*L*QA*alpha*eV*gA*lambda)/C1;
% G19=- (4*K2*L*QV*alpha*eV*gA*lambda)/C1;
% G20=- (4*K2*L*Qvad*alpha*eA*gA*lambda)/C1;
% G21=- 4*C1*KA*L*QA*alpha*eA*gA;
% G22=+ 4*C1*KA*L*QLV*alpha*eA*gA;
% G23=- 4*C1*KA*L*QA*alpha*eV*gA;
% G24=+ 4*C1*KA*L*QV*alpha*eV*gA;
% G25=+ 4*C1*KA*L*Qvad*alpha*eA*gA;
% G26=+ 4*L*QA_dot*alpha*eA*eV*gA^2;
% G27=- 4*L*QV_dot*alpha*eA*eV*gA^2;
% G28=+ 4*K1*KA*L*QA*alpha*eA*gA;
% G29=- 4*K1*KA*L*QA_ref*alpha*eA*gA;
% 
% 
% GG1 = [G1 G2 G3 G4 G5 G6 G7 G8 G9 G10 G11 G12 G13 G14 G15 G16 G17 G18 G19 G20];
% GG2 = [G21 G22 G23 G24 G25 G26 G27 G28 G29];
% GGG1 = sum(GG1) + sum(GG2);
% 
% GGG2=((4*C1*QLV*alpha*eA^2*gA^2 + C1*Qvad^4*a1^2*eA^2*gA^2*gLV + C1*Qvad^2*b1^2*eA^2*gA^2*gLV + 4*K2*L*QA_ref_dot*alpha*gLV*lambda - 4*C1^2*KA*L*QA_ref_dot*alpha*gLV - 4*C1*Qvad^2*a2*alpha*eA^2*gA^2*gLV + 2*C1*Qvad^3*a1*b1*eA^2*gA^2*gLV ...
%     + 4*C1*L*QA_dot*alpha*eA^2*gA^2*gLV - 4*C1*L*QLV_dot*alpha*eA^2*gA^2*gLV - 4*C1*Qvad*alpha*b2*eA^2*gA^2*gLV - 4*K1*K2*L*QA*alpha*gLV*lambda + 4*K1*K2*L*QA_ref*alpha*gLV*lambda + 4*C1*L*QA_ref_ddot*alpha*eA*gA*gLV ...
%     + 4*C1^2*K1*KA*L*QA*alpha*gLV - 4*C1^2*K1*KA*L*QA_ref*alpha*gLV + 4*K2*L*QA*alpha*eA*gA*gLV*lambda - 4*K2*L*QLV*alpha*eA*gA*gLV*lambda + 4*K2*L*QA*alpha*eV*gA*gLV*lambda - 4*K2*L*QV*alpha*eV*gA*gLV*lambda ...
%     - 4*K2*L*Qvad*alpha*eA*gA*gLV*lambda - 4*C1^2*KA*L*QA*alpha*eA*gA*gLV + 4*C1^2*KA*L*QLV*alpha*eA*gA*gLV - 4*C1^2*KA*L*QA*alpha*eV*gA*gLV + 4*C1^2*KA*L*QV*alpha*eV*gA*gLV + 4*C1^2*KA*L*Qvad*alpha*eA*gA*gLV ...
%     + 4*C1*L*QA_dot*alpha*eA*eV*gA^2*gLV - 4*C1*L*QV_dot*alpha*eA*eV*gA^2*gLV + 4*C1*K1*KA*L*QA*alpha*eA*gA*gLV - 4*C1*K1*KA*L*QA_ref*alpha*eA*gA*gLV)/(C1*gLV));

== matlab function HMC/IBS_LVAD/Subsystem1/PUMP/VAD1 ==
  data: Q output; Q_pre input; W input; DP input
function  Q = fcn(Q_pre,W,DP)
alpha=3.241e-6;
a1=6.657e-5;
a2=-1.807;
b1=0.001263;
b2=0.1433;
L= 6;
dt = 1e-4;

R=-(a1.*W+a2).*Q_pre-(b1.*W+b2);

Q_dot = (1/L)*(alpha.*W.^2-DP-R.*Q_pre);

Q = Q_pre + Q_dot*dt;

== matlab function HMC/IBS_LVAD/Subsystem1/Subsystem/Pressures Flows and Volumes1/MATLAB Function ==
  data: u input; y output; HR input
function y = fcn(u,HR)

tbeatlol =60/HR;
y = mod(u,tbeatlol);
end

== matlab function HMC/Subsystem/MATLAB Function9 ==
  data: pwm input; output output; pwm_delayed input
function output = fcn(pwm,pwm_delayed)
a=0.4;
b=0.1;
check = pwm-pwm_delayed;
if a > pwm & b < abs(check)
    output = 1;
else
    output = 0;
end

== matlab function HMC/MATLAB Function9 ==
  data: C input; per output; t input; tt_pre input; tt output
function [per,tt] = fcn(C,t,tt_pre)


if C==1
       
    tt=t;
    
else
    
    tt=tt_pre;
    
end 

per = t-tt;

== matlab function HMC/Subsystem1/MATLAB Function2 ==
  data: g1h input; g2h input; g3h input; g4h input; g5h input; g6h input; g1h_dot output; g2h_dot output; g3h_dot output; g4h_dot output; g5h_dot output; g6h_dot output; Qvad input; phi2 output; phi3 output; u output; Qvad_dot input; DP input; DP_dot input; DV input; W input; i input; k1 input; k2 input; k3 input; gam1 input; gam2 input; gam3 input; gam4 input; gam5 input; gam6 input; W_dot output; i_dot output
function [g1h_dot, g2h_dot, g3h_dot, g4h_dot, g5h_dot,g6h_dot, phi2, phi3, u,W_dot,i_dot] = fcn(g1h, g2h, g3h, g4h, g5h, g6h, Qvad, Qvad_dot, DP, DP_dot, DV, W, i, k1, k2, k3,gam1,gam2,gam3,gam4,gam5,gam6)

x1=DV; x2=W; x3=i;

J=0.293e-3; L=1.44e-3;
K=72.4e-3; Rbf=2.399e+9; Rgp= 0.48;
a_w=1.59e-6; a_P=3.625e-6;
tau1=44.9e-6; tau2=0.3e-3;

f1=2*Qvad-(2/Rbf)*DP ; f2=-tau1*sign(W)-a_P*DP;

f1dot=2*Qvad_dot-(2/Rbf)*DP_dot; f2dot=-a_P*DP_dot; 


g1h_dot =-(x1*gam1*(f1 + x1*k1))/g1h;
 
g2h_dot =x2*gam2*(x2 + (f1 + x1*k1)/g1h);
 
g3h_dot =-(gam3*(x2 + (f1 + x1*k1)/g1h)*(f2 + g2h*(x2 + (f1 + x1*k1)/g1h) + (f1dot - k1*(x1*k1 - g1h*(x2 + (f1 + x1*k1)/g1h)))/g1h + k2*(x2 + (f1 + x1*k1)/g1h) + g1h*x1 - (g2h*(f1 + x1*k1))/g1h + (x1*gam1*(f1 + x1*k1)^2)/g1h^3))/g3h;

g4h_dot =x2*gam4*(x3 + (f2 + g2h*(x2 + (f1 + x1*k1)/g1h) + (f1dot - k1*(x1*k1 - g1h*(x2 + (f1 + x1*k1)/g1h)))/g1h + k2*(x2 + (f1 + x1*k1)/g1h) + g1h*x1 - (g2h*(f1 + x1*k1))/g1h + (x1*gam1*(f1 + x1*k1)^2)/g1h^3)/g3h);

g5h_dot =x3*gam5*(x3 + (f2 + g2h*(x2 + (f1 + x1*k1)/g1h) + (f1dot - k1*(x1*k1 - g1h*(x2 + (f1 + x1*k1)/g1h)))/g1h + k2*(x2 + (f1 + x1*k1)/g1h) + g1h*x1 - (g2h*(f1 + x1*k1))/g1h + (x1*gam1*(f1 + x1*k1)^2)/g1h^3)/g3h);

g6h_dot =-(gam6*(x3 + (f2 + g2h*(x2 + (f1 + x1*k1)/g1h) + (f1dot - k1*(x1*k1 - g1h*(x2 + (f1 + x1*k1)/g1h)))/g1h + k2*(x2 + (f1 + x1*k1)/g1h) + g1h*x1 - (g2h*(f1 + x1*k1))/g1h + (x1*gam1*(f1 + x1*k1)^2)/g1h^3)/g3h)*(g3h*(x2 + (f1 + x1*k1)/g1h) + g4h*(x2 + (f1 + x1*k1)/g1h) - (g2h*(k2*(x2 + (f1 + x1*k1)/g1h) - g3h*(x3 + (f2 + g2h*(x2 + (f1 + x1*k1)/g1h) + (f1dot - k1*(x1*k1 - g1h*(x2 + (f1 + x1*k1)/g1h)))/g1h + k2*(x2 + (f1 + x1*k1)/g1h) + g1h*x1 - (g2h*(f1 + x1*k1))/g1h + (x1*gam1*(f1 + x1*k1)^2)/g1h^3)/g3h) + g1h*x1) - f2dot + k2*(k2*(x2 + (f1 + x1*k1)/g1h) - g3h*(x3 + (f2 + g2h*(x2 + (f1 + x1*k1)/g1h) + (f1dot - k1*(x1*k1 - g1h*(x2 + (f1 + x1*k1)/g1h)))/g1h + k2*(x2 + (f1 + x1*k1)/g1h) + g1h*x1 - (g2h*(f1 + x1*k1))/g1h + (x1*gam1*(f1 + x1*k1)^2)/g1h^3)/g3h) + g1h*x1) + g1h*(x1*k1 - g1h*(x2 + (f1 + x1*k1)/g1h)) - x2*gam2*(x2 + (f1 + x1*k1)/g1h)^2 + (g2h*(f1dot - k1*(x1*k1 - g1h*(x2 + (f1 + x1*k1)/g1h))))/g1h + (x1^2*gam1*(f1 + x1*k1))/g1h + (x2*gam2*(x2 + (f1 + x1*k1)/g1h)*(f1 + x1*k1))/g1h + (g2h*x1*gam1*(f1 + x1*k1)^2)/g1h^3)/g3h + g5h*(x3 + (f2 + g2h*(x2 + (f1 + x1*k1)/g1h) + (f1dot - k1*(x1*k1 - g1h*(x2 + (f1 + x1*k1)/g1h)))/g1h + k2*(x2 + (f1 + x1*k1)/g1h) + g1h*x1 - (g2h*(f1 + x1*k1))/g1h + (x1*gam1*(f1 + x1*k1)^2)/g1h^3)/g3h) + k3*(x3 + (f2 + g2h*(x2 + (f1 + x1*k1)/g1h) + (f1dot - k1*(x1*k1 - g1h*(x2 + (f1 + x1*k1)/g1h)))/g1h + k2*(x2 + (f1 + x1*k1)/g1h) + g1h*x1 - (g2h*(f1 + x1*k1))/g1h + (x1*gam1*(f1 + x1*k1)^2)/g1h^3)/g3h) - (g4h*(f1 + x1*k1))/g1h - (g5h*(f2 + g2h*(x2 + (f1 + x1*k1)/g1h) + (f1dot - k1*(x1*k1 - g1h*(x2 + (f1 + x1*k1)/g1h)))/g1h + k2*(x2 + (f1 + x1*k1)/g1h) + g1h*x1 - (g2h*(f1 + x1*k1))/g1h + (x1*gam1*(f1 + x1*k1)^2)/g1h^3))/g3h + (gam3*(x2 + (f1 + x1*k1)/g1h)*(f2 + g2h*(x2 + (f1 + x1*k1)/g1h) + (f1dot - k1*(x1*k1 - g1h*(x2 + (f1 + x1*k1)/g1h)))/g1h + k2*(x2 + (f1 + x1*k1)/g1h) + g1h*x1 - (g2h*(f1 + x1*k1))/g1h + (x1*gam1*(f1 + x1*k1)^2)/g1h^3)^2)/g3h^3))/g6h;

phi2 =-(f1 + x1*k1)/g1h;

phi3 =-(f2 + g2h*(x2 + (f1 + x1*k1)/g1h) + (f1dot - k1*(x1*k1 - g1h*(x2 + (f1 + x1*k1)/g1h)))/g1h + k2*(x2 + (f1 + x1*k1)/g1h) + g1h*x1 - (g2h*(f1 + x1*k1))/g1h + (x1*gam1*(f1 + x1*k1)^2)/g1h^3)/g3h;
 
u =-(g3h*(x2 + (f1 + x1*k1)/g1h) + g4h*(x2 + (f1 + x1*k1)/g1h) - (g2h*(k2*(x2 + (f1 + x1*k1)/g1h) - g3h*(x3 + (f2 + g2h*(x2 + (f1 + x1*k1)/g1h) + (f1dot - k1*(x1*k1 - g1h*(x2 + (f1 + x1*k1)/g1h)))/g1h + k2*(x2 + (f1 + x1*k1)/g1h) + g1h*x1 - (g2h*(f1 + x1*k1))/g1h + (x1*gam1*(f1 + x1*k1)^2)/g1h^3)/g3h) + g1h*x1) - f2dot + k2*(k2*(x2 + (f1 + x1*k1)/g1h) - g3h*(x3 + (f2 + g2h*(x2 + (f1 + x1*k1)/g1h) + (f1dot - k1*(x1*k1 - g1h*(x2 + (f1 + x1*k1)/g1h)))/g1h + k2*(x2 + (f1 + x1*k1)/g1h) + g1h*x1 - (g2h*(f1 + x1*k1))/g1h + (x1*gam1*(f1 + x1*k1)^2)/g1h^3)/g3h) + g1h*x1) + g1h*(x1*k1 - g1h*(x2 + (f1 + x1*k1)/g1h)) - x2*gam2*(x2 + (f1 + x1*k1)/g1h)^2 + (g2h*(f1dot - k1*(x1*k1 - g1h*(x2 + (f1 + x1*k1)/g1h))))/g1h + (x1^2*gam1*(f1 + x1*k1))/g1h + (x2*gam2*(x2 + (f1 + x1*k1)/g1h)*(f1 + x1*k1))/g1h + (g2h*x1*gam1*(f1 + x1*k1)^2)/g1h^3)/g3h + g5h*(x3 + (f2 + g2h*(x2 + (f1 + x1*k1)/g1h) + (f1dot - k1*(x1*k1 - g1h*(x2 + (f1 + x1*k1)/g1h)))/g1h + k2*(x2 + (f1 + x1*k1)/g1h) + g1h*x1 - (g2h*(f1 + x1*k1))/g1h + (x1*gam1*(f1 + x1*k1)^2)/g1h^3)/g3h) + k3*(x3 + (f2 + g2h*(x2 + (f1 + x1*k1)/g1h) + (f1dot - k1*(x1*k1 - g1h*(x2 + (f1 + x1*k1)/g1h)))/g1h + k2*(x2 + (f1 + x1*k1)/g1h) + g1h*x1 - (g2h*(f1 + x1*k1))/g1h + (x1*gam1*(f1 + x1*k1)^2)/g1h^3)/g3h) - (g4h*(f1 + x1*k1))/g1h - (g5h*(f2 + g2h*(x2 + (f1 + x1*k1)/g1h) + (f1dot - k1*(x1*k1 - g1h*(x2 + (f1 + x1*k1)/g1h)))/g1h + k2*(x2 + (f1 + x1*k1)/g1h) + g1h*x1 - (g2h*(f1 + x1*k1))/g1h + (x1*gam1*(f1 + x1*k1)^2)/g1h^3))/g3h + (gam3*(x2 + (f1 + x1*k1)/g1h)*(f2 + g2h*(x2 + (f1 + x1*k1)/g1h) + (f1dot - k1*(x1*k1 - g1h*(x2 + (f1 + x1*k1)/g1h)))/g1h + k2*(x2 + (f1 + x1*k1)/g1h) + g1h*x1 - (g2h*(f1 + x1*k1))/g1h + (x1*gam1*(f1 + x1*k1)^2)/g1h^3)^2)/g3h^3)/g6h;


t=sign(W)*tau1+W*tau2;

W_dot=(1/J)*(-t+K*i-a_P*DP);

i_dot=(1/L)*(-K*W-Rgp*i+u);

== matlab function HMC/DV_calc/MATLAB Function3 ==
  data: P2 input; Pp2 input; V2 output; P3 input; V3 output; Pp3 input; DV output
function [V2,V3,DV] = fcn(P2,Pp2,P3,Pp3)



r = 0.09/2;
A = pi*r^2;

rho = 997;
g = 9.81;
eh = rho*g/A;

Ph2=P2-Pp2;
Ph3=P3-Pp3;

V2=Ph2/eh;
V3=Ph3/eh;

DV=V2-V3;
